simulink model "pll_simulation"  (R2018b)
settings: Solver=VariableStepAuto  StartTime=0.0  StopTime=50  MaxStep=5e-4  RelTol=1e-3
settings Model: Creator=dvarx  LastModifiedBy=dvarx

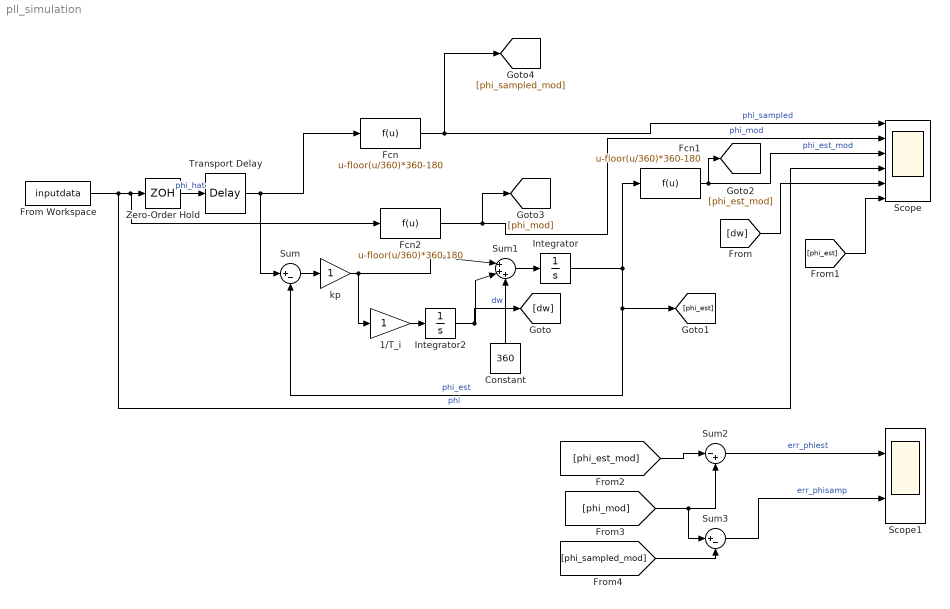
== system pll_simulation ==
  1/T_i : Gain
  Constant : Constant  Value=360
  Fcn : Fcn  Expr=u-floor(u/360)*360-180
  Fcn1 : Fcn  Expr=u-floor(u/360)*360-180
  Fcn2 : Fcn  Expr=u-floor(u/360)*360-180
  From Workspace : FromWorkspace  VariableName=inputdata  SampleTime=0
  Integrator : Integrator
  Integrator2 : Integrator
  Scope : Scope  NumInputPorts=6
  Scope1 : Scope  NumInputPorts=2
  Sum : Sum  Inputs=|+-
  Sum1 : Sum  Inputs=|+++
  Sum2 : Sum  Inputs=|-+
  Sum3 : Sum  Inputs=|+-
  Transport Delay : TransportDelay  DelayTime=1e-3
  Zero-Order Hold : ZeroOrderHold  SampleTime=0.010
  kp : Gain
  wires:
  From Workspace/1 -> Fcn2/1, Zero-Order Hold/1, Scope/4  "phi"
  Sum1/1 -> Integrator/1
  Integrator/1 -> [phi_est], Sum/2, Fcn1/1  "phi_est"
  Sum/1 -> kp/1
  kp/1 -> 1/T_i/1, Sum1/1
  Constant/1 -> Sum1/3
  1/T_i/1 -> Integrator2/1
  Integrator2/1 -> [dw], Sum1/2  "dw"
  Fcn/1 -> [phi_sampled_mod], Scope/1  "phi_sampled"
  Fcn1/1 -> [phi_est_mod], Scope/3  "phi_est_mod"
  Fcn2/1 -> [phi_mod], Scope/2  "phi_mod"
  [dw] -> Scope/5
  [phi_est] -> Scope/6
  Sum2/1 -> Scope1/1  "err_phiest"
  Sum3/1 -> Scope1/2  "err_phisamp"
  [phi_mod] -> Sum3/1, Sum2/2
  [phi_est_mod] -> Sum2/1
  [phi_sampled_mod] -> Sum3/2
  Zero-Order Hold/1 -> Transport Delay/1  "phi_hat"
  Transport Delay/1 -> Sum/1, Fcn/1
